simulink model "product_demo"  (Simulink 6.3)
settings: Solver=ode45  StartTime=0.0  StopTime=10.0  RelTol=1e-3
settings Model: LastModifiedBy=Ms1

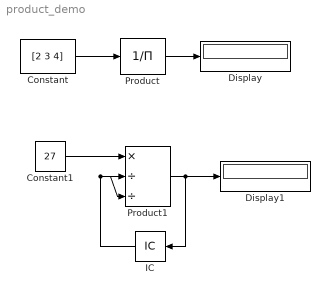
== system product_demo ==
  Constant : Constant  Value=[2 3 4]
  Constant1 : Constant  Value=27
  Display : Display
  Display1 : Display
  IC : InitialCondition  Orientation=left
  Product : Product  Inputs=/  SaturateOnIntegerOverflow=on  InputSameDT=on
  Product1 : Product  Inputs=*//  SaturateOnIntegerOverflow=on  InputSameDT=on
  wires:
  Constant/1 -> Product/1
  Product/1 -> Display/1
  Product1/1 -> Display1/1, IC/1
  Constant1/1 -> Product1/1
  IC/1 -> Product1/2, Product1/3
